simulink model "TwoSpecies"  (Simulink 6.6)
settings: Solver=ode45  StartTime=0.0  StopTime=10  RelTol=1e-3
settings Model: Creator=MXKana  LastModifiedBy=mxkana

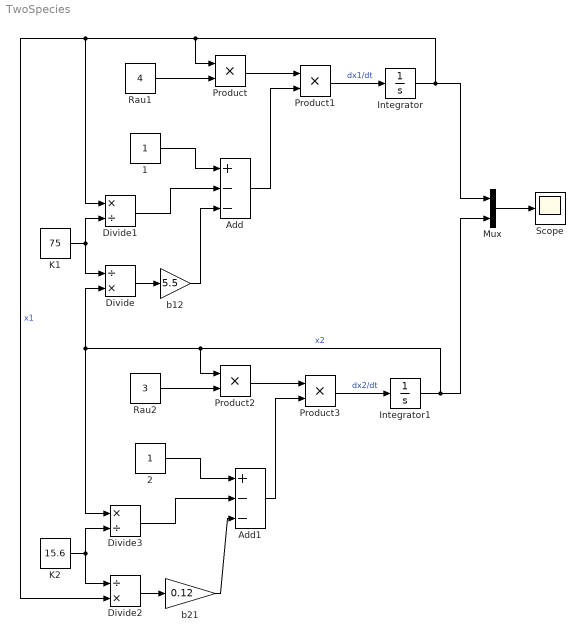
== system TwoSpecies ==
  1 : Constant
  2 : Constant
  Add : Sum  Inputs=+--  OutScaling=2^-10
  Add1 : Sum  Inputs=+--  OutScaling=2^-10
  Divide : Product  Inputs=/*  OutScaling=2^-10
  Divide1 : Product  Inputs=*/  OutScaling=2^-10
  Divide2 : Product  Inputs=/*  OutScaling=2^-10
  Divide3 : Product  Inputs=*/  OutScaling=2^-10
  Integrator : Integrator  InitialCondition=1
  Integrator1 : Integrator  InitialCondition=1
  K1 : Constant  Value=75
  K2 : Constant  Value=15.6
  Mux : Mux  Inputs=2
  Product{,1..3} (4 alike) : Product  RndMeth=Zero
  Rau1 : Constant  Value=4
  Rau2 : Constant  Value=3
  Scope : Scope
      settings: YMin=0  YMax=20
  b12 : Gain  Gain=5.5
  b21 : Gain  Gain=0.12
  wires:
  Product/1 -> Product1/1
  Product1/1 -> Integrator/1  "dx1/dt"
  Rau1/1 -> Product/2
  1/1 -> Add/1
  Integrator/1 -> Product/1, Divide1/1, Divide2/2, Mux/1  "x1"
  K1/1 -> Divide/1, Divide1/2
  Divide/1 -> b12/1
  b12/1 -> Add/3
  Divide1/1 -> Add/2
  Add/1 -> Product1/2
  Product2/1 -> Product3/1
  Product3/1 -> Integrator1/1  "dx2/dt"
  Rau2/1 -> Product2/2
  2/1 -> Add1/1
  Integrator1/1 -> Product2/1, Divide/2, Divide3/1, Mux/2  "x2"
  K2/1 -> Divide2/1, Divide3/2
  Divide2/1 -> b21/1
  b21/1 -> Add1/3
  Divide3/1 -> Add1/2
  Add1/1 -> Product3/2
  Mux/1 -> Scope/1
